simulink model "Traffic_light_system"  (R2020b)
settings: Solver=VariableStepAuto  StartTime=0.0  StopTime=10.0  RelTol=1e-3
settings Model: Creator=Varun  LastModifiedBy=Varun

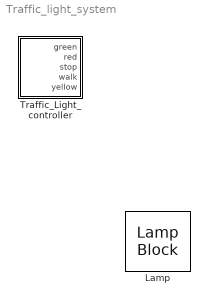
== system Traffic_light_system ==
  Lamp : LampBlock
  Traffic_Light_controller : Stateflow chart  TreatAsAtomicUnit=on

== stateflow chart Traffic_light_system/Traffic_Light_controller ==
  state TrafficGo
    entry:
    red=0;
    yellow=0;
    green=1;
    walk=0;
    stop=1;
  state TrafficCaution
    entry:
    red=0;
    yellow=1;
    green=0;
    walk=0;
    stop=1;
  state TrafficStop
    entry:
    red=1;
    yellow=0;
    green=0;
    walk=1;
    stop=0;
  (default) -> TrafficGo
  data: green output; red output; stop output; walk output; yellow output
